simulink model "current_controller"  (R2019b)
settings: Solver=VariableStepAuto  StartTime=0.0  StopTime=10.0  RelTol=1e-3
InitFcn:
  | R = 1.6
  | 
  | Lq = 0.0225
  | 
  | Ld = 0.01975
  | 
  | 
  | PM  = 75*3.14/180
  | 
  | Wc = 392
  | 
  | Ti = 0.01
  | 
  | 
  | PI_q = tand(PM - 90 + atand((Wc*Lq)/R) + atand(Wc*Ti));
  | 
  | Ki = (Wc * sqrt(((R)^2)+((Wc*Lq)^2)) * sqrt(1 + (Wc*Ti)^2)/sqrt(1+(PI_q)^2));
  | 
  | Kp = (PI_q * Ki)/Wc;
  | 
  | 
  | PI_d = tand(PM - 90 + atand((Wc*Ld)/R) + atand(Wc*Ti));
  | 
  | Ki_d = (Wc * sqrt(((R)^2)+((Wc*Ld)^2)) * sqrt(1 + (Wc*Ti)^2)/sqrt(1+(PI_d)^2));
  | 
  | Kp_d = (PI_d * Ki_d)/Wc;
settings Model: Creator=kanth  LastModifiedBy=kanth

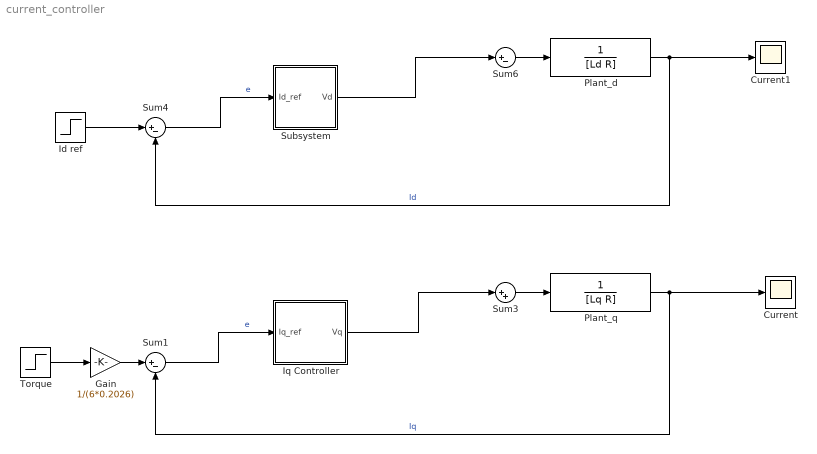
== system current_controller ==
  Current : Scope
  Current1 : Scope
  Gain : Gain  Gain=1/(6*0.2026)
  Id ref : Step  Time=10  After=10  SampleTime=0
  Iq Controller : Subsystem
  Plant_d : TransferFcn  Denominator=[Ld R]
  Plant_q : TransferFcn  Denominator=[Lq R]
  Subsystem : Subsystem
  Sum1 : Sum  Inputs=|+-
  Sum3 : Sum  Inputs=|++
  Sum4 : Sum  Inputs=|+-
  Sum6 : Sum  Inputs=|+-
  "Torque " : Step  After=10  SampleTime=0
  wires:
  "Torque "/1 -> Gain/1
  Sum3/1 -> Plant_q/1
  Plant_q/1 -> Sum1/2, Current/1  "Iq"
  Gain/1 -> Sum1/1
  Plant_d/1 -> Sum4/2, Current1/1  "Id"
  Sum6/1 -> Plant_d/1
  Id ref/1 -> Sum4/1
  Sum1/1 -> Iq Controller/1(Iq_ref)  "e"
  Iq Controller/1(Vq) -> Sum3/1
  Sum4/1 -> Subsystem/1(Id_ref)  "e"
  Subsystem/1(Vd) -> Sum6/1

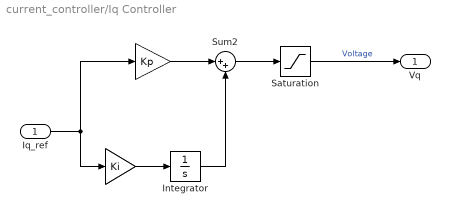
== system current_controller/Iq Controller ==
  Iq_ref : Inport
  " " : Gain  Gain=Kp
  "  " : Gain  Gain=Ki
  Integrator : Integrator  LimitOutput=on  UpperSaturationLimit=150  LowerSaturationLimit=-150
  Saturation : Saturate  UpperLimit=170  LowerLimit=-170
  Sum2 : Sum  Inputs=|++
  Vq : Outport
  wires:
  "  "/1 -> Integrator/1
  Sum2/1 -> Saturation/1
  " "/1 -> Sum2/1
  Integrator/1 -> Sum2/2
  Iq_ref/1 -> "  "/1, " "/1
  Saturation/1 -> Vq/1  "Voltage"

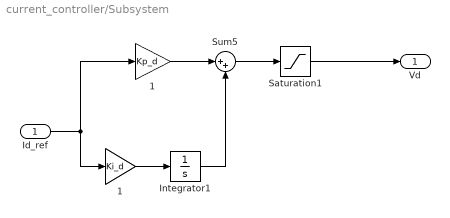
== system current_controller/Subsystem ==
  Id_ref : Inport
  "  1" : Gain  Gain=Ki_d
  " 1" : Gain  Gain=Kp_d
  Integrator1 : Integrator  LimitOutput=on  UpperSaturationLimit=8  LowerSaturationLimit=-8
  Saturation1 : Saturate  UpperLimit=10  LowerLimit=-10
  Sum5 : Sum  Inputs=|++
  Vd : Outport
  wires:
  "  1"/1 -> Integrator1/1
  Id_ref/1 -> " 1"/1, "  1"/1
  Integrator1/1 -> Sum5/2
  Sum5/1 -> Saturation1/1
  Saturation1/1 -> Vd/1
  " 1"/1 -> Sum5/1
